simulink model "untitled"  (R2019b)
settings: Solver=VariableStepAuto  StartTime=0.0  StopTime=10.0  RelTol=1e-3
values from neighbouring files (symbols this model uses):
  A = [0 1 ... (first row only)    [Untitled.m]
  Azart = A-B*K    [Untitled.m]
  B = [0;1/M]    [Untitled.m]
  Bzart = zeros(size(B))    [Untitled.m]
  C = [1 0]    [Untitled.m]
  K = inv(R)*B'*P    [Untitled.m]
  x0 = [10;10]    [Untitled.m]
settings Model: Creator=patti  LastModifiedBy=patti

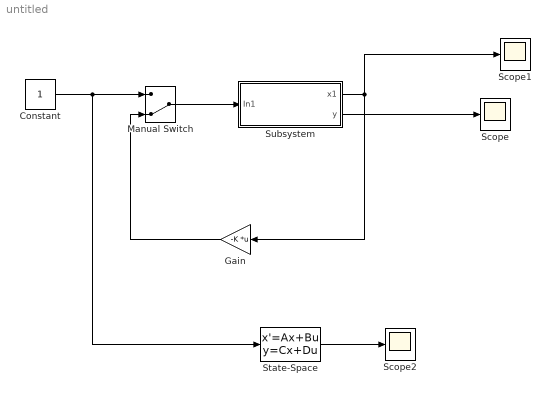
== system untitled ==
  Constant : Constant
  Gain : Gain  Gain=-K  Multiplication=Matrix(K*u)
  Manual Switch : ManualSwitch  CurrentSetting=0
  Scope : Scope
  Scope1 : Scope
  Scope2 : Scope
  State-Space : StateSpace  A=Azart  B=Bzart  C=eye(2)  D=[0;0]  InitialCondition=x0
  Subsystem : Subsystem
  wires:
  Constant/1 -> State-Space/1, Manual Switch/1
  Manual Switch/1 -> Subsystem/1(In1)
  Subsystem/1("x1 ") -> Scope1/1, Gain/1
  Gain/1 -> Manual Switch/2
  Subsystem/2("y ") -> Scope/1
  State-Space/1 -> Scope2/1

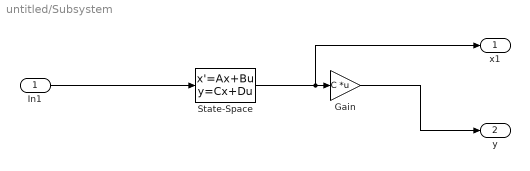
== system untitled/Subsystem ==
  In1 : Inport
  Gain : Gain  Gain=C  Multiplication=Matrix(K*u)
  State-Space : StateSpace  A=A  B=B  C=eye(2)  D=[0;0]  InitialCondition=x0
  "x1 " : Outport
  "y " : Outport  Port=2
  wires:
  In1/1 -> State-Space/1
  State-Space/1 -> "x1 "/1, Gain/1
  Gain/1 -> "y "/1
